simulink model "simCRM_IdealWindEst"  (R2016b)
settings: Solver=ode5  StartTime=0.0  StopTime=SimConfig.EndTime  FixedStep=SimConfig.SampleTime  RelTol=1e-3
libraries: Actuators_Block x1, lib_Sim_CRM x1, Controllers x1, Lidar_IdealWind x1, Sensors_Block x1
settings Model: Creator=cava_da  LastModifiedBy=cava_da
settings DataIOCC: Decimation=SimConfig.Logging.DecimationFactor  SaveFormat=StructureWithTime  ReturnWorkspaceOutputs=on
settings OptimizationCC: ExpressionDepthLimit=2147483647  InitFltsAndDblsToZero=on  LifeSpan=inf
settings DebuggingCC: UnderspecifiedInitializationDetection=Classic  MergeDetectMultiDrivingBlocksExec=none  SolverPrmCheckMsg=warning  FcnCallInpInsideContextMsg=warning  StateNameClashWarn=warning  SFUnexpectedBacktrackingDiag=warning  SFNoUnconditionalDefaultTransitionDiag=warning  SFExecutionAtInitializationDiag=none
settings HardwareCC: ProdBitPerPointer=32  ProdBitPerSizeT=32  ProdBitPerPtrDiffT=32  ProdLargestAtomicFloat=None  ProdIntDivRoundTo=Undefined  ProdEndianess=Unspecified  ProdWordSize=32  ProdHWDeviceType=32-bit Generic
settings ModelReferenceCC: PropagateSignalLabelsOutOfModel=off
settings SFSimCC: SimUseLocalCustomCode=on
settings RTWCC: RTWUseLocalCustomCode=on
settings GRTTargetCC: TargetLangStandard=C89/C90 (ANSI)  CombineOutputUpdateFcns=off  GRTInterface=on
settings ConfigComp: CovMetricSettings=dw  CovHtmlReporting=on  CovSaveCumulativeToWorkspaceVar=on  CovSaveSingleToWorkspaceVar=on

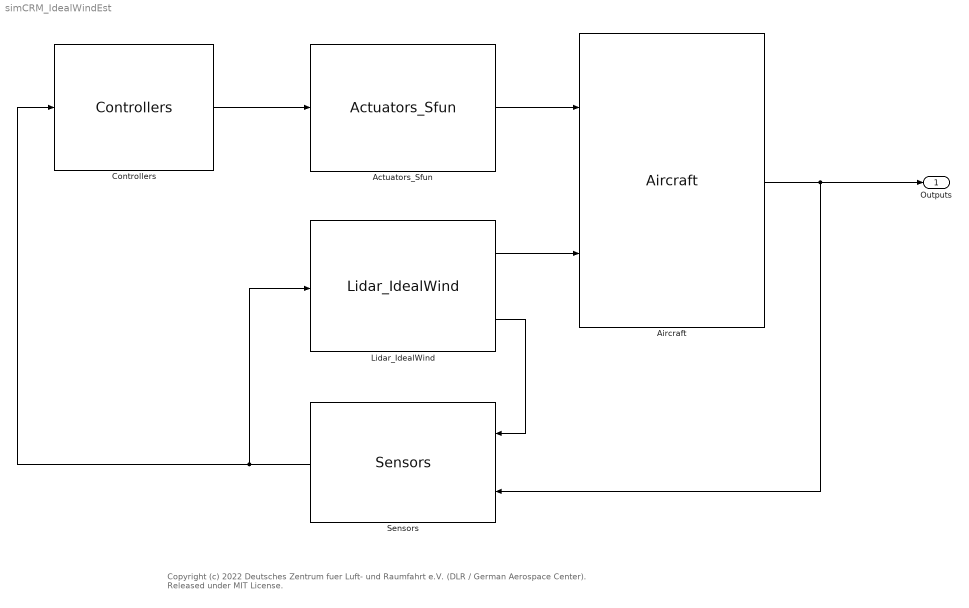
== system simCRM_IdealWindEst ==
  note: Copyright (c) 2022 Deutsches Zentrum fuer Luft- und Raumfahrt e.V. (DLR / German Aerospace Center). Released under MIT License.
  Actuators_Sfun : Actuators_Block/Actuators_Sfun  SystemSampleTime=-1
  Aircraft : lib_Sim_CRM/Aircraft  modelName=CRM.Aircraft
  Controllers : Controllers/Controllers  SystemSampleTime=-1
  Lidar_IdealWind : Lidar_IdealWind/Lidar_IdealWind  SystemSampleTime=-1
  Sensors : Sensors_Block/Sensors  SystemSampleTime=-1
  Outputs : Outport
  wires:
  Lidar_IdealWind/1 -> Aircraft/2
  Aircraft/1 -> Sensors/2, Outputs/1
  Lidar_IdealWind/2 -> Sensors/1
  Sensors/1 -> Controllers/1, Lidar_IdealWind/1
  Controllers/1 -> Actuators_Sfun/1
  Actuators_Sfun/1 -> Aircraft/1
